simulink model "PC_MSFS_STATION"  (R2021b)
settings: Solver=FixedStepAuto  StartTime=0.0  StopTime=700  FixedStep=0.03  RelTol=1e-3
undefined symbols (not defined in the file): DiscIntNeverNeededParam, f, MODEL, MODEL_INI
libraries: SimConnectToolbox x13, simulink x5, instrumentlib x3
(part 2 of 2)

== matlab function PC_MSFS_STATION/CONTROL/CONTROL UPDATE ==
  data: CONTROL_IN input; CONTROL output Bus: CONTROL_Bus; STATE input; ALTITUDE input
function CONTROL = CONTROL_UPDATE(CONTROL_IN, STATE, ALTITUDE)
% COPY CONTROL BUS
CONTROL = CONTROL_IN;
CONTROL.PARAM.SIM_TIME = CONTROL.PARAM.SIM_TIME + CONTROL.PARAM.SAMPLING_TIME;
curr_sim_time = CONTROL.PARAM.SIM_TIME;
deltat = CONTROL.PARAM.SAMPLING_TIME;
flight_status = CONTROL.PARAM.FLIGHT_STATUS;
timer = CONTROL.PARAM.TIMER;

%--------------------------------------------------------------------------
% CONTROL PARAMETERS
%--------------------------------------------------------------------------
% Nominal Control Parameters
kyd = CONTROL.PARAM.NAV_D_1;

% Navigation Variables
altitude = ALTITUDE;
altitude_control = CONTROL.PARAM.ALTITUDE;
rho = altitude + 20.902e6;

% Safety Filters (CBF)
time_Safe = CONTROL.PARAM.TIME_SAFE;
dist_Threshold = CONTROL.PARAM.DIST_THRESHOLD;
dist_Critical = CONTROL.PARAM.DIST_CRITICAL;
wp_Threshold_Flag = CONTROL.PARAM.WP_THRESHOLD;
time_WP = CONTROL.PARAM.WP_TIMER;

CBF_const = CONTROL.PARAM.CBF_CONST;
CBF_active = CONTROL.PARAM.CBF_ACTIVE_FLAG;
h = CONTROL.PARAM.CBF_H;
psi = CONTROL.PARAM.CBF_PSI;

% Extra Parameters
tau_max = CONTROL.PARAM.TAU_MAX;
dist_Goal = CONTROL.PARAM.DIST_GOAL;

fval_qp = CONTROL.PARAM.FVAL;
exitval_qp = CONTROL.PARAM.EXITVAL;

%--------------------------------------------------------------------------
% CONTROL TARGETS
%--------------------------------------------------------------------------
wp_index = CONTROL.TARGET.WP_INDEX;
simu_end = CONTROL.TARGET.SIMU_END;
target_latitude = CONTROL.TARGET.LATITUDE*pi/180;
target_longitude = CONTROL.TARGET.LONGITUDE*pi/180;
snom = CONTROL.TARGET.VELOCITY;
%--------------------------------------------------------------------------
% SYSTEM CURRENT STATE
%--------------------------------------------------------------------------
% Update Current State
y1 = STATE(1);
y2 = STATE(2);
vy1 = STATE(3);
vy2 = STATE(4);

% FLIGHT STATUS 0 = INITIALIZATION
if flight_status == 0
    % VIRTUAL NOMINAL CONTROLLER (tau1, tau2)
    tau1_nom_PD = - kyd*(vy1 - 0);
    tau2_nom_PD = - kyd*(vy2 - 0);
    tau1_applied = tau1_nom_PD;
    tau2_applied = tau2_nom_PD;
    
    if abs(tau1_applied) >= tau_max
        tau1_applied = sign(tau1_applied)*tau_max;
    else
        tau1_applied = tau1_applied;
    end
    
    if abs(tau2_applied) >= tau_max
        tau2_applied = sign(tau2_applied)*tau_max;
    else
        tau2_applied = tau2_applied;
    end
    if curr_sim_time >= 10 && CONTROL.TARGET.LATITUDE ~= 0
        flight_status = 1;
        timer = 0;
    end 

elseif flight_status == 1

    altitude = altitude_control;
    rho = altitude + 20.902e6;
    tau1_nom_PD = - kyd*(vy1 - 0);
    tau2_nom_PD = - kyd*(vy2 - 0);
    tau1_applied = tau1_nom_PD;
    tau2_applied = tau2_nom_PD;

    if abs(tau1_applied) >= tau_max
        tau1_applied = sign(tau1_applied)*tau_max;
    else
        tau1_applied = tau1_applied;
    end
    
    if abs(tau2_applied) >= tau_max
        tau2_applied = sign(tau2_applied)*tau_max;
    else
        tau2_applied = tau2_applied;
    end
    if curr_sim_time >= 30 
        flight_status = 2;
        timer = 0;
    end
elseif flight_status == 2
    % ON FLIGHT
    %--------------------------------------------------------------------------
    % DERIVATIVE (D) CONTROL
    %--------------------------------------------------------------------------
    altitude = altitude_control;
    rho = altitude + 20.902e6; 
    timer = timer + deltat;
    time_WP = time_WP + deltat;

    wp1 = rho*cos(target_latitude)*cos(target_longitude);
    wp2 = rho*cos(target_latitude)*sin(target_longitude);

    % UPDATE SAFETY FILTER ACTIVE
    if ((y1 - wp1)^2 + (y2 - wp2)^2 < dist_Threshold^2)
        if wp_Threshold_Flag == 0
            % System just crossed the threshold
            wp_Threshold_Flag = 1; % Only enters here once
            time_WP = 0; % Start timer
        end
        if (time_WP <= time_Safe)
            % Safe time hasn't expired
            CBF_active = 1;
        else
            % Safe time has expired
            CBF_active = 0; % System can now reach waypoint
        end
    end
    
    % UPDATE TARGET WAYPOINT
    if ((y1 - wp1)^2 < dist_Goal^2)&&((y2 - wp2)^2 < dist_Goal^2)
        % UPDATE WAYPOINT INDEX
%         wp_index = wp_index + 1;
        % UPDATE SAFETY FILTER PARAMETERS
        CBF_active = 0;
        wp_Threshold_Flag = 0;
        %simu_end = 1;
        flight_status = 3;

%         if (wp_index >= 3) % Total WP + 1
%             simu_end = 1;
%             CBF_active = 0;
%             flight_status = 3;
%             wp_index = 2; % Final WP index
%         end
    end

    % UPDATE TARGET VELOCITY
    if simu_end == 0
        % System Quadrant
        pos1_PD = wp1 - y1;
        pos2_PD = wp2 - y2;

        if pos1_PD >=0
            % First or fourth quadrant
            if pos2_PD >=0
                %First quadrant
                theta_PD = atan(abs(pos2_PD)/abs(pos1_PD));
            else
                % Fourth quadrant
%                 theta_PD = 2*pi - atan(abs(pos2_PD)/abs(pos1_PD));
                theta_PD = - atan(abs(pos2_PD)/abs(pos1_PD));
            end
        else
            % Second or third quadrant
            if pos2_PD >=0
                % Second quadrant
                theta_PD = pi - atan(abs(pos2_PD)/abs(pos1_PD));
            else
                % Third quadrant
                theta_PD = pi + atan(abs(pos2_PD)/abs(pos1_PD));
            end
        end

        % New target velocity
        vs1_PD = snom*cos(theta_PD);
        vs2_PD = snom*sin(theta_PD);

        % VIRTUAL NOMINAL CONTROLLER (tau1, tau2)
        tau1_nom_PD = - kyd*(vy1 - vs1_PD);
        tau2_nom_PD = - kyd*(vy2 - vs2_PD);

        if (CBF_active == 1)
            % SAFETY FILTERS
            h = (y1 - wp1)^2 + (y2 - wp2)^2 - dist_Critical^2;
            hdot = 2*(y1 - wp1)*vy1 + 2*(y2 - wp2)*vy2;
            psi = hdot + CBF_const*h;

            % QUAD PROG COMPONENTS
            A1_qp = 2*(y1 - wp1);
            A2_qp = 2*(y2 - wp2);
            b1_qp = 2*(vy1^2 + vy2^2) + CBF_const*hdot + CBF_const*psi;
            A_qp = -[A1_qp, A2_qp];
            b_qp = [b1_qp];
            H_qp = [1, 0; 0, 1];
            f_qp = -2*[tau1_nom_PD; tau2_nom_PD];
            x0_qp = [tau1_nom_PD; tau2_nom_PD];
            option_qp = optimoptions('quadprog','Algorithm','active-set','Display','None');
            [tau_applied, fval_qp, exitval_qp] = quadprog(H_qp, double(f_qp), A_qp, b_qp,[],[],[],[],x0_qp,option_qp);
            tau1_applied = tau_applied(1);
            tau2_applied = tau_applied(2);
        else
            tau1_applied = tau1_nom_PD;
            tau2_applied = tau2_nom_PD; 
        end

    else
        % VIRTUAL NOMINAL CONTROLLER (tau1, tau2)
        tau1_applied = - kyd*(vy1 - 0);
        tau2_applied = - kyd*(vy2 - 0);
        tau1_nom_PD = tau1_applied;
        tau2_nom_PD = tau2_applied;
    end

    if abs(tau1_applied) >= tau_max
        tau1_applied = sign(tau1_applied)*tau_max;
    else
        tau1_applied = tau1_applied;
    end

    if abs(tau2_applied) >= tau_max
        tau2_applied = sign(tau2_applied)*tau_max;
    else
        tau2_applied = tau2_applied;
    end

    if simu_end == 1
        flight_status = 3;
    end 
else
     % END OF MISSION
    tau1_nom_PD = - kyd*(vy1 - 0);
    tau2_nom_PD = - kyd*(vy2 - 0);
    tau1_applied = tau1_nom_PD;
    tau2_applied = tau2_nom_PD;
    
    if abs(tau1_applied) >= tau_max
        tau1_applied = sign(tau1_applied)*tau_max;
    else
        tau1_applied = tau1_applied;
    end

    if abs(tau2_applied) >= tau_max
        tau2_applied = sign(tau2_applied)*tau_max;
    else
        tau2_applied = tau2_applied;
    end
    if simu_end == 0
        altitude = altitude_control;
    end
    rho = altitude + 20.902e6;
    
end


%%%%%%%%%%%%%%%%%%%%%%%%%%%%%%%%%%%%%%%%%%%%%%%%%%%%%%%%%%%%%%%%%%%%%%%%%%%
% OUTPUT BUS
%%%%%%%%%%%%%%%%%%%%%%%%%%%%%%%%%%%%%%%%%%%%%%%%%%%%%%%%%%%%%%%%%%%%%%%%%%%
CONTROL.TARGET.WP_INDEX = wp_index;
CONTROL.TARGET.SIMU_END = simu_end;
CONTROL.OUTPUT.TAU1 = tau1_applied;
CONTROL.OUTPUT.TAU2 = tau2_applied;

CONTROL.PARAM.FLIGHT_STATUS = flight_status;
CONTROL.PARAM.ALTITUDE = altitude;
CONTROL.PARAM.RHO = rho;
CONTROL.PARAM.TIMER = timer;

CONTROL.PARAM.WP_THRESHOLD = wp_Threshold_Flag;
CONTROL.PARAM.WP_TIMER = time_WP;
CONTROL.PARAM.CBF_ACTIVE_FLAG = CBF_active;

CONTROL.PARAM.FVAL = fval_qp;
CONTROL.PARAM.EXITVAL = exitval_qp;

CONTROL.PARAM.CBF_H = h;
CONTROL.PARAM.CBF_PSI = psi;
CONTROL.OUTPUT.TAU1_NOM = tau1_nom_PD;
CONTROL.OUTPUT.TAU2_NOM = tau2_nom_PD;
return

== matlab function PC_MSFS_STATION/SYSTEM/UNICYCLE MODEL ==
  data: STATE input; STATE_DERIVATIVE output; MODEL_IN input; MODEL output Bus: MODEL_Bus
function [STATE_DERIVATIVE,MODEL] = SO_UNICYCLE_MODEL(STATE, MODEL_IN)
% COPY MODEL BUS
MODEL = MODEL_IN;
%--------------------------------------------------------------------------
% SO UNICYCLE PARAMETERS
%--------------------------------------------------------------------------
dist_p = MODEL.PARAM.DISP_P;
flight_status = MODEL.PARAM.FLIGHT_STATUS;
%--------------------------------------------------------------------------
% EVALUATE FLIGHT STATUS
%--------------------------------------------------------------------------
% if flight_status == 0
% %     % INITIALIZATION
% %     theta_long = MODEL.INPUT.LONGITUDE;
% %     phi_lat = MODEL.INPUT.LATITUDE;
% %     altitude = MODEL.INPUT.ALTITUDE;
% %     rho = altitude + 20.902e6;
% %     % Displaced Point Dynamics Y = {y1, y2, vy1, vy2}
% %     y1 = rho*cos(phi_lat)*cos(theta_long);
% %     y2 = rho*cos(phi_lat)*sin(theta_long);
% %     vy1 = 0;
% %     vy2 = 0;
% %     % Center of Mass Dynamics X = {x1, x2, s, theta, omega}
% %     s = 0;
% %     theta = 0;
% %     omega = 0;
% %     x1 = y1 - dist_p*cos(theta);
% %     x2 = y2 - dist_p*sin(theta);
% % NEW APPROACH
% %     altitude = 2*10e2;
% %     rho = altitude + 20.902e6;
%     % Displaced Point Dynamics Y = {y1, y2, vy1, vy2}
%     y1 = STATE(1);
%     y2 = STATE(2);
%     vy1 = STATE(3);
%     vy2 = STATE(4);
%     % Center of Mass Dynamics X = {x1, x2, s, theta, omega}
%     s = STATE(5);
%     theta = STATE(6);
%     omega = STATE(7);
%     x1 = y1 - dist_p*cos(theta);
%     x2 = y2 - dist_p*sin(theta);
%     % Update Latitude and Longitude
%     altitude = MODEL.INPUT.ALTITUDE;
%     rho = altitude + 20.902e6;
%     if y1 >=0
%         % First or fourth quadrant
%         if y2 >=0
%             %First quadrant
%             theta_long = atan(abs(y2)/abs(y1));
%         else
%             % Fourth quadrant
%             %         theta_long = 2*pi - atan(abs(y2)/abs(y1));
%             theta_long = - atan(abs(y2)/abs(y1));
%         end
%     else
%         % Second or third quadrant
%         if y2 >=0
%             % Second quadrant
%             theta_long = pi - atan(abs(y2)/abs(y1));
%         else
%             % Third quadrant
%             theta_long = pi + atan(abs(y2)/abs(y1));
%         end
%     end
%     phi_lat = acos(y1/(rho*cos(theta_long)));
%     
% elseif flight_status == 1
% %     % TAKE OFF
% %     theta_long = MODEL.INPUT.LONGITUDE;
% %     phi_lat = MODEL.INPUT.LATITUDE;
% %     altitude = 2*10e2;
% %     rho = altitude + 20.902e6;
% %     % Displaced Point Dynamics Y = {y1, y2, vy1, vy2}
% %     y1 = rho*cos(phi_lat)*cos(theta_long);
% %     y2 = rho*cos(phi_lat)*sin(theta_long);
% %     vy1 = 0;
% %     vy2 = 0;
% %     % Center of Mass Dynamics X = {x1, x2, s, theta, omega}
% %     s = 0;
% %     theta = 0;
% %     omega = 0;
% %     x1 = y1 - dist_p*cos(theta);
% %     x2 = y2 - dist_p*sin(theta);
%     % NEW APPROACH
% %     altitude = 2*10e2;
% %     rho = altitude + 20.902e6;
%     % Displaced Point Dynamics Y = {y1, y2, vy1, vy2}
%     y1 = STATE(1);
%     y2 = STATE(2);
%     vy1 = STATE(3);
%     vy2 = STATE(4);
%     % Center of Mass Dynamics X = {x1, x2, s, theta, omega}
%     s = STATE(5);
%     theta = STATE(6);
%     omega = STATE(7);
%     x1 = y1 - dist_p*cos(theta);
%     x2 = y2 - dist_p*sin(theta);
%     % Update Latitude and Longitude
%     altitude = MODEL.INPUT.ALTITUDE;
%     rho = altitude + 20.902e6;
%     if y1 >=0
%         % First or fourth quadrant
%         if y2 >=0
%             %First quadrant
%             theta_long = atan(abs(y2)/abs(y1));
%         else
%             % Fourth quadrant
%             %         theta_long = 2*pi - atan(abs(y2)/abs(y1));
%             theta_long = - atan(abs(y2)/abs(y1));
%         end
%     else
%         % Second or third quadrant
%         if y2 >=0
%             % Second quadrant
%             theta_long = pi - atan(abs(y2)/abs(y1));
%         else
%             % Third quadrant
%             theta_long = pi + atan(abs(y2)/abs(y1));
%         end
%     end
%     phi_lat = acos(y1/(rho*cos(theta_long)));
% else
    % ON FLIGHT
    %--------------------------------------------------------------------------
    % STATE VARIABLES
    %--------------------------------------------------------------------------
    % Displaced Point Dynamics Y = {y1, y2, vy1, vy2}
    y1 = STATE(1);
    y2 = STATE(2);
    vy1 = STATE(3);
    vy2 = STATE(4);
    % Center of Mass Dynamics X = {x1, x2, s, theta, omega}
    s = STATE(5);
    theta = STATE(6);
    omega = STATE(7);
    x1 = y1 - dist_p*cos(theta);
    x2 = y2 - dist_p*sin(theta);
    % Update Latitude and Longitude
    altitude = MODEL.INPUT.ALTITUDE;
    rho = altitude + 20.902e6;
    if y1 >=0
        % First or fourth quadrant
        if y2 >=0
            %First quadrant
            theta_long = atan(abs(y2)/abs(y1));
        else
            % Fourth quadrant
            %         theta_long = 2*pi - atan(abs(y2)/abs(y1));
            theta_long = - atan(abs(y2)/abs(y1));
        end
    else
        % Second or third quadrant
        if y2 >=0
            % Second quadrant
            theta_long = pi - atan(abs(y2)/abs(y1));
        else
            % Third quadrant
            theta_long = pi + atan(abs(y2)/abs(y1));
        end
    end
    phi_lat = acos(y1/(rho*cos(theta_long)));
% end
%--------------------------------------------------------------------------
% HEADING CONTROL
%--------------------------------------------------------------------------
% CHANGE OF FRAME FROM XYZ TO NED
sinPOS_Lat = sin(phi_lat);
cosPOS_Lat = cos(phi_lat);
sinPOS_Long = sin(theta_long);
cosPOS_Long = cos(theta_long);

Iner_to_NED = zeros(3,3);
Iner_to_NED(1,1) = - sinPOS_Lat*cosPOS_Long;
Iner_to_NED(2,1) = - sinPOS_Long;
Iner_to_NED(3,1) = - cosPOS_Lat*cosPOS_Long;
Iner_to_NED(1,2) = - sinPOS_Lat*sinPOS_Long;
Iner_to_NED(2,2) = cosPOS_Long;
Iner_to_NED(3,2) = - cosPOS_Lat*sinPOS_Long;
Iner_to_NED(1,3) = cosPOS_Lat;
Iner_to_NED(2,3) = 0;
Iner_to_NED(3,3) = - sinPOS_Lat;

NED_vy = Iner_to_NED*[vy1;vy2;0];
NED_vy1 = NED_vy(1); % NORTH
NED_vy2 = NED_vy(2); % EAST
heading_NED = atan2(NED_vy2,NED_vy1);
heading = atan2(vy2,vy1);
%--------------------------------------------------------------------------
% INPUTS
%--------------------------------------------------------------------------
tau1 = MODEL.INPUT.TAU1;
tau2 = MODEL.INPUT.TAU2;
%--------------------------------------------------------------------------
% STATE EQUATIONS
%--------------------------------------------------------------------------
y1dot = vy1;
y2dot = vy2;
y1ddot = tau1;
y2ddot = tau2;
sdot = -omega^2*dist_p + tau1*cos(theta) + tau2*sin(theta);
thetadot = omega;
omegadot = 1/dist_p*(omega*s - tau1*sin(theta) + tau2*cos(theta));
%--------------------------------------------------------------------------
% STATE DERIVATIVES
%--------------------------------------------------------------------------
STATE_DERIVATIVE = [y1dot; y2dot; y1ddot; y2ddot; sdot; thetadot; omegadot];
%%%%%%%%%%%%%%%%%%%%%%%%%%%%%%%%%%%%%%%%%%%%%%%%%%%%%%%%%%%%%%%%%%%%%%%%%%%
% OUTPUT BUS
%%%%%%%%%%%%%%%%%%%%%%%%%%%%%%%%%%%%%%%%%%%%%%%%%%%%%%%%%%%%%%%%%%%%%%%%%%%
MODEL.STATE = [y1 ; y2 ; vy1 ; vy2 ; s ; theta ; omega];
MODEL.OUTPUT.X1 = x1;
MODEL.OUTPUT.X2 = x2;
MODEL.OUTPUT.X = sqrt(x1^2 + x2^2);
MODEL.OUTPUT.Y = sqrt(y1^2 + y2^2);
MODEL.OUTPUT.LATITUDE = phi_lat;
MODEL.OUTPUT.LONGITUDE = theta_long;
MODEL.OUTPUT.HEADING = heading; 
MODEL.OUTPUT.HEADING_NED = heading_NED; 
return
